simulink model "exer_3_2"  (Simulink 7.5)
settings: Solver=ode45  StartTime=0.0  StopTime=1000  RelTol=1e-3
values from neighbouring files (symbols this model uses):
  gama1 = 5    [EXER_3_1.m]    (also in EXER_3_2.m = 1; EXER_3_3.m = 1)
  gama2 = 5    [EXER_3_1.m]    (also in EXER_3_2.m = 1; EXER_3_3.m = 1)
  UC = 1    [EXER_3_1.m]    (also in EXER_3_2.m; EXER_3_3.m)
settings Model: Creator=jijo  LastModifiedBy=morteza

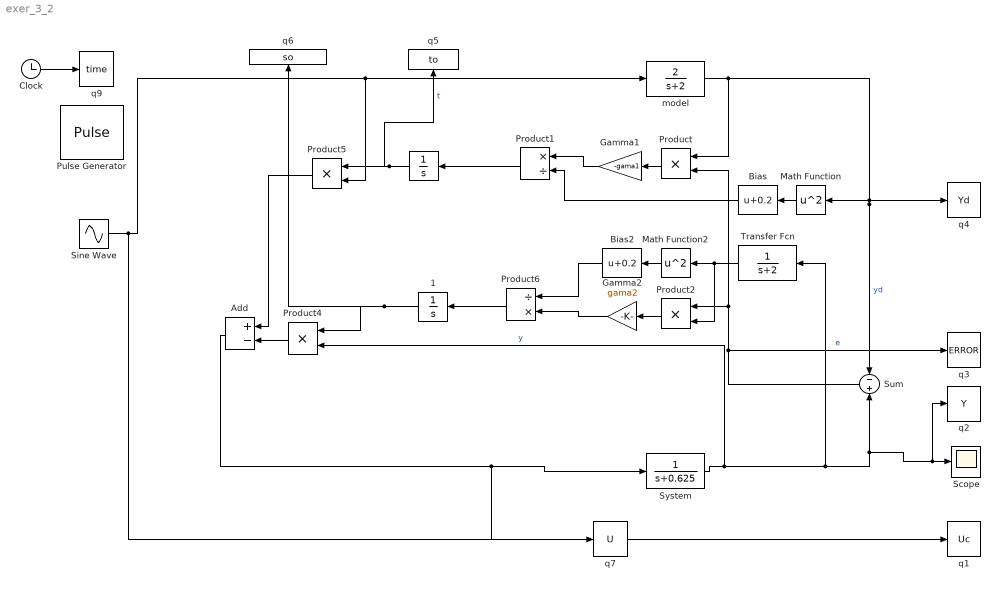
== system exer_3_2 ==
  " " : Integrator
  " 1" : Integrator
  Add : Sum  Inputs=+-  OutDataType=fixdt(1, 16)  OutScaling=2^-10
  Bias : Bias  Bias=0.2
  Bias2 : Bias  Bias=0.2
  Clock : Clock
      settings: Decimation=10
  Gamma1 : Gain  Gain=-gama1  ParameterDataType=fixdt(1, 16)  ParameterScaling=2^0  OutDataType=fixdt(1, 16)  OutScaling=2^0
  Gamma2 : Gain  Gain=gama2  ParameterDataType=fixdt(1, 16)  ParameterScaling=2^0  OutDataType=fixdt(1, 16)  OutScaling=2^0
  Math Function : Math  Operator=square  OutDataType=fixdt(1, 16)  OutScaling=2^0  SaturateOnIntegerOverflow=on
  Math Function2 : Math  Operator=square  OutDataType=fixdt(1, 16)  OutScaling=2^0  SaturateOnIntegerOverflow=on
  Product{,2,4..5} (4 alike) : Product  OutDataType=fixdt(1, 16)  OutScaling=2^0  RndMeth=Zero
  Product1 : Product  Inputs=*/  OutDataType=fixdt(1, 16)  OutScaling=2^0  RndMeth=Zero
  Product6 : Product  Inputs=/*  OutDataType=fixdt(1, 16)  OutScaling=2^0  RndMeth=Zero
  Pulse Generator : DiscretePulseGenerator  PulseType=Time based  Amplitude=UC  Period=200  PulseWidth=50  PhaseDelay=0  SampleTime=1
  Scope : Scope
      settings: YMin=-2000  YMax=2500
  Sine Wave : Sin  Amplitude=1  Bias=0  Frequency=5  Phase=0  Samples=10  SampleTime=0  Offset=0
  Sum : Sum  Inputs=-+  OutDataType=fixdt(1, 16)  OutScaling=2^0
  System : TransferFcn  Denominator=[1 0.625]
  Transfer Fcn : TransferFcn  Denominator=[1 2]
  model : TransferFcn  Numerator=[2]  Denominator=[1 2]
  q1 : ToWorkspace  VariableName=Uc  SampleTime=-1  SaveFormat=Array
  q2 : ToWorkspace  VariableName=Y  SampleTime=-1  SaveFormat=Array
  q3 : ToWorkspace  VariableName=ERROR  SampleTime=-1  SaveFormat=Array
  q4 : ToWorkspace  VariableName=Yd  SampleTime=-1  SaveFormat=Array
  q5 : ToWorkspace  VariableName=to  SampleTime=-1  SaveFormat=Array
  q6 : ToWorkspace  VariableName=so  SampleTime=-1  SaveFormat=Array
  q7 : ToWorkspace  VariableName=U  SampleTime=-1  SaveFormat=Array
  q9 : ToWorkspace  VariableName=time  SampleTime=-1  SaveFormat=Array
  wires:
  model/1 -> Product/1, q4/1, Math Function/1, Sum/1  "yd"
  System/1 -> Sum/2, Scope/1, q2/1, Transfer Fcn/1, Product4/2  "y"
  Product/1 -> Gamma1/1
  Sum/1 -> q3/1, Product/2, Product2/1  "e"
  " "/1 -> Product5/1, q5/1  "t"
  Product2/1 -> Gamma2/1
  " 1"/1 -> q6/1, Product4/1
  Add/1 -> System/1, q7/1
  Clock/1 -> q9/1
  Product4/1 -> Add/2
  Math Function/1 -> Bias/1
  Bias/1 -> Product1/2
  Gamma1/1 -> Product1/1
  Product1/1 -> " "/1
  Transfer Fcn/1 -> Math Function2/1, Product2/2
  Math Function2/1 -> Bias2/1
  Bias2/1 -> Product6/1
  Gamma2/1 -> Product6/2
  Product6/1 -> " 1"/1
  Product5/1 -> Add/1
  Sine Wave/1 -> q1/1, model/1, Product5/2
